simulink library "HEMERO"  (Simulink 3.00)
values from neighbouring files (symbols this model uses):
  K1 = 0.5    [ejh64.m]    (also in ejh65.m)
  K2 = 0.8    [ejh64.m]    (also in ejh65.m)
  x_camino = 0:0.01:10    [ejh64.m]    (also in ejh65.m)
  y_camino = x_camino.^2    [ejh64.m]    (also in ejh65.m)
undefined symbols (not defined in the file or in its folder): magnitude, nonlinear
libraries: simulink_extras x12, HEMERO x9, simulink3 x6, dspstat x4
(part 3 of 9)

== system HEMERO/Robots móviles/Control de robots móviles/Métodos basados en Teoría de Control/Seguimiento de trayectorias ==
  Ejemplos : Subsystem
  Seguimiento de trayectorias (Control lineal con escalado de velocidad) : Subsystem  mask(Seguimiento de trayectorias (control lineal y escalado en velocidad)){b=, d=, x_inicial=, y_inicial=, phi_inicial=, x_r_inicial=, y_r_inicial=, phi_r_inicial=}
      mask prompts: b "Parámetro beta:"; d "Parámetro delta:"; x_inicial "Coordenada x inicial del robot:"; y_inicial "Coordenada y inicial del robot:"; phi_inicial "Valor inicial de la orientación del robot (rad):"; x_r_inicial "Coordenada x inicial de la referencia:"; y_r_inicial "Coordenada y inicial de la referencia:"; phi_r_inicial "Orientación inicial de la referencia (rad):"
      mask help:
      | Este bloque permite simular una estrategia de control lineal con "escalado en velocidad" para el seguimiento de trayectorias. A la entrada se dispone de las velocidades lineal y angular de referencia. Se supone un cierto modelo para el vehículo.
      | El usuario puede modificar este bloque para introducir como referencia las coordenadas (x,y) y la orientación deseadas.
  Seguimiento de trayectorias (Control lineal) : Subsystem  mask(Seguimiento de trayectorias empleando una ley de control lineal){K1=, K2=, K3=, x_inicial=, y_inicial=, phi_inicial=, x_r_inicial=, y_r_inicial=, phi_r_inicial=}
      mask prompts: K1 "Parámetro K1:"; K2 "Parámetro K2:"; K3 "Parámetro K3:"; x_inicial "Coordenada x inicial del robot:"; y_inicial "Coordenada y inicial del robot:"; phi_inicial "Valor inicial de la orientación del robot (rad):"; x_r_inicial "Coordenada x inicial de la referencia:"; y_r_inicial "Coordenada y inicial de la referencia:"; phi_r_inicial "Orientación inicial de la referencia (rad):"
      mask help:
      | Este bloque permite simular una estrategia de control lineal para el seguimiento de trayectorias. A la entrada se dispone de las velocidades lineal y angular de referencia. Se supone un cierto modelo para el vehículo.
      | El usuario puede modificar este bloque para introducir como referencia las coordenadas (x,y) y la orientación deseadas.
  Seguimiento de trayectorias (Control no lineal) : Subsystem  mask(Seguimiento de trayectorias empleando una ley de control no lineal){b=, d=, K2=, x_inicial=, y_inicial=, phi_inicial=, x_r_inicial=, y_r_inicial=, phi_r_inicial=}
      mask prompts: b "Parámetro beta:"; d "Parámetro delta:"; K2 "Parámetro K2:"; x_inicial "Coordenada x inicial del robot:"; y_inicial "Coordenada y inicial del robot:"; phi_inicial "Valor inicial de la orientación del robot (rad):"; x_r_inicial "Coordenada x inicial de la referencia:"; y_r_inicial "Coordenada y inicial de la referencia:"; phi_r_inicial "Orientación inicial de la referencia (rad):"
      mask help:
      | Este bloque permite simular una estrategia de control no lineal para el seguimiento de trayectorias. A la entrada se dispone de las velocidades lineal y angular de referencia. Se supone un cierto modelo para el vehículo.
      | El usuario puede modificar este bloque para introducir como referencia las coordenadas (x,y) y la orientación deseadas.

== system HEMERO/Robots móviles/Modelos cinemáticos inversos/Modelo inverso Bicicleta/Cálculo de phi ==
  x ' : Inport  Port=1  PortWidth=-1  SampleTime=-1  DataType=auto
      settings: SignalType=auto
  y ' : Inport  Port=2  PortWidth=-1  SampleTime=-1  DataType=auto
      settings: SignalType=auto
  MATLAB Fcn : MATLABFcn  MATLABFcn=auxinv  OutputWidth=1  OutputSignalType=auto
  Mux : Mux  Inputs=2
      settings: DisplayOption=none
  phi : Outport  Port=1
  wires:
  Mux/1 -> MATLAB Fcn/1
  y '/1 -> Mux/2
  x '/1 -> Mux/1
  MATLAB Fcn/1 -> phi/1

== system HEMERO/Robots móviles/Modelos cinemáticos inversos/Modelo inverso Config. Síncrona/Cálculo de phi ==
  x ' : Inport  Port=1  PortWidth=-1  SampleTime=-1  DataType=auto
      settings: SignalType=auto
  y ' : Inport  Port=2  PortWidth=-1  SampleTime=-1  DataType=auto
      settings: SignalType=auto
  MATLAB Fcn : MATLABFcn  MATLABFcn=auxinv  OutputWidth=1  OutputSignalType=auto
  Mux : Mux  Inputs=2
      settings: DisplayOption=none
  phi : Outport  Port=1
  wires:
  Mux/1 -> MATLAB Fcn/1
  y '/1 -> Mux/2
  x '/1 -> Mux/1
  MATLAB Fcn/1 -> phi/1

== system HEMERO/Robots móviles/Modelos cinemáticos inversos/Modelo inverso Guiado Diferencial/Cálculo de phi ==
  x ' : Inport  Port=1  PortWidth=-1  SampleTime=-1  DataType=auto
      settings: SignalType=auto
  y ' : Inport  Port=2  PortWidth=-1  SampleTime=-1  DataType=auto
      settings: SignalType=auto
  MATLAB Fcn : MATLABFcn  MATLABFcn=auxinv  OutputWidth=1  OutputSignalType=auto
  Mux : Mux  Inputs=2
      settings: DisplayOption=none
  phi : Outport  Port=1
  wires:
  Mux/1 -> MATLAB Fcn/1
  y '/1 -> Mux/2
  x '/1 -> Mux/1
  MATLAB Fcn/1 -> phi/1

== system HEMERO/Robots móviles/Modelos cinemáticos inversos/Modelo inverso Triciclo Clasico/Cálculo de phi ==
  x ' : Inport  Port=1  PortWidth=-1  SampleTime=-1  DataType=auto
      settings: SignalType=auto
  y ' : Inport  Port=2  PortWidth=-1  SampleTime=-1  DataType=auto
      settings: SignalType=auto
  MATLAB Fcn : MATLABFcn  MATLABFcn=auxinv  OutputWidth=1  OutputSignalType=auto
  Mux : Mux  Inputs=2
      settings: DisplayOption=none
  phi : Outport  Port=1
  wires:
  MATLAB Fcn/1 -> phi/1
  x '/1 -> Mux/1
  y '/1 -> Mux/2
  Mux/1 -> MATLAB Fcn/1

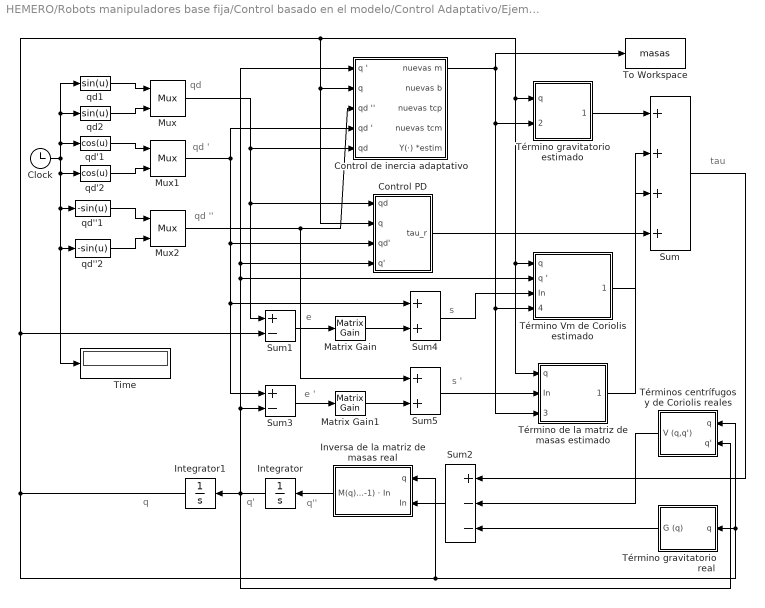
== system HEMERO/Robots manipuladores base fija/Control basado en el modelo/Control Adaptativo/Ejemplos/Ejemplo H.5.5 ==
  note: q''
  note: q'
  note: q
  note: tau
  note: e
  note: e '
  note: s
  note: s '
  note: qd
  note: qd '
  note: qd ''
  Clock : Clock
      settings: DisplayTime=off  Decimation=10
  Control PD : Subsystem  mask(Controlador PD){A=[2.5 0;0 2.5], Kv=[10 0;0 10]}
      mask prompts: A "Introduzca la matriz A:"; Kv "Introduzca la matriz Kv:"
      mask help: Calcula el par tau_r correspondiente a la técnica del par computado usando un controlador PD.
  Control de inercia adaptativo : Subsystem  mask(Técnica del par computado con control adaptativo){dyn=[0 0 0 0 0 30 1 0 0 0 0 0 0 0 0 0 1 0 0 0;0 1 0 0 0 100 1 0 0 0 0 0 0 0 0 0 1 0 0 0], gamma=[20 0 zeros(1,6); 0 20 zeros(1,6); zeros(6,8)], a=[2.5 0;0 2.5], grav=[0 -9.81 0], m_inicial=[30 100], b_inicial=[0 0], tcp_inicial=[0 0], tcm_inicial=[0 0]}
      mask prompts: dyn "Matriz de parámetros cinemáticos y dinámicos:"; gamma "Matriz gamma:"; a "Matriz A:"; grav "Vector aceleración de la gravedad:"; m_inicial "Estimaciones de las masas:"; b_inicial "Estimaciones de las fricciones viscosas:"; tcp_inicial "Estimaciones de las fricciones de Coulomb (rotación +):"; tcm_inicial "Estimaciones de las fricciones de Coulomb (rotación -):"
  Integrator : Integrator  Orientation=left  ExternalReset=none  InitialConditionSource=internal  InitialCondition=[0;0]  LimitOutput=off  UpperSaturationLimit=inf  LowerSaturationLimit=-inf  ShowSaturationPort=off  ShowStatePort=off  AbsoluteTolerance=auto
  Integrator1 : Integrator  Orientation=left  ExternalReset=none  InitialConditionSource=internal  InitialCondition=[0; 0]  LimitOutput=off  UpperSaturationLimit=inf  LowerSaturationLimit=-inf  ShowSaturationPort=off  ShowStatePort=off  AbsoluteTolerance=auto
  Inversa de la matriz de masas real : Subsystem  Orientation=left  mask(Inversa de la matriz de masas){dyn=[0 0 0 0 0 0.8 1 0 0 0 0 0 0 0 0 0 1 0 0 0;0 1 0 0 0 2.3 1 0 0 0 0 0 0 0 0 0 1 0 0 0]}
      mask prompts: dyn "Matriz de parámetros cinemáticos y dinámicos:"
      mask help: Este bloque calcula el producto de la inversa de la matriz de masas por el vector columna In que se le pasa como entrada.
  Matrix Gain : simulink3/Math/Matrix Gain  K=[2.5 0;0 2.5]
  Matrix Gain1 : simulink3/Math/Matrix Gain  K=[2.5 0;0 2.5]
  Mux : Mux  Inputs=2
      settings: DisplayOption=none
  Mux1 : Mux  Inputs=2
      settings: DisplayOption=none
  Mux2 : Mux  Inputs=2
      settings: DisplayOption=none
  Sum : Sum  Inputs=++++  SaturateOnIntegerOverflow=on
  Sum1 : Sum  Inputs=+-  SaturateOnIntegerOverflow=on
  Sum2 : Sum  Orientation=left  Inputs=+--  SaturateOnIntegerOverflow=on
  Sum3 : Sum  Inputs=+-  SaturateOnIntegerOverflow=on
  Sum4 : Sum  Inputs=++  SaturateOnIntegerOverflow=on
  Sum5 : Sum  Inputs=++  SaturateOnIntegerOverflow=on
  Time : Display
      settings: Format=short
  To Workspace : ToWorkspace  VariableName=masas  SampleTime=-1  SaveFormat=Matrix
  Término gravitatorio estimado : Subsystem  mask(Término gravitatorio estimado){dyn=[0 0 0 0 0 30 1 0 0 0 0 0 0 0 0 0 1 0 0 0;0 1 0 0 0 100 1 0 0 0 0 0 0 0 0 0 1 0 0 0], grav=[0 -9.81 0]}
      mask prompts: dyn "Matriz inicial de parámetros cinemáticos y dinámicos:"; grav "Vector aceleración de la gravedad:"
      mask help: Este bloque calcula el par correspondiente al término gravitatorio. Dispone de una entrada para proporcionarle las estimaciones de las masas en cada instante.
      mask Display:
      | plot([0.05 0.95],[0.05 0.95])
      | plot([0.8 0.95],[0.7 0.95])
      | plot([0.7 0.95],[0.8 0.95])
  Término gravitatorio real : Subsystem  Orientation=left  mask(Término gravitatorio){dyn=[0 0 0 0 0 0.8 1 0 0 0 0 0 0 0 0 0 1 0 0 0;0 1 0 0 0 2.3 1 0 0 0 0 0 0 0 0 0 1 0 0 0], grav=[0 -9.81 0]}
      mask prompts: dyn "Matriz de parámetros cinemáticos y dinámicos:"; grav "Vector aceleración de la gravedad:"
      mask help: Este bloque calcula el par correspondiente al término gravitatorio.
  Término Vm de Coriolis estimado : Subsystem  mask(Término estimado asociado a la matriz de masas){dyn=[0 0 0 0 0 30 1 0 0 0 0 0 0 0 0 0 1 0 0 0;0 1 0 0 0 100 1 0 0 0 0 0 0 0 0 0 1 0 0 0]}
      mask prompts: dyn "Matriz inicial de parámetros cinemáticos y dinámicos:"
      mask help: Este bloque calcula el par correspondiente al término en el que aparece la matriz de masas. Dispone de una entrada para proporcionarle las estimaciones de las masas en cada instante.
      mask Display:
      | plot([0.05 0.95],[0.05 0.95])
      | plot([0.8 0.95],[0.7 0.95])
      | plot([0.7 0.95],[0.8 0.95])
  Término de la matriz de masas estimado : Subsystem  mask(Término estimado asociado a la matriz de masas){dyn=[0 0 0 0 0 30 1 0 0 0 0 0 0 0 0 0 1 0 0 0;0 1 0 0 0 100 1 0 0 0 0 0 0 0 0 0 1 0 0 0]}
      mask prompts: dyn "Matriz inicial de parámetros cinemáticos y dinámicos:"
      mask help: Este bloque calcula el par correspondiente al término en el que aparece la matriz de masas. Dispone de una entrada para proporcionarle las estimaciones de las masas en cada instante.
      mask Display:
      | plot([0.05 0.95],[0.05 0.95])
      | plot([0.8 0.95],[0.7 0.95])
      | plot([0.7 0.95],[0.8 0.95])
  Términos centrífugos y de Coriolis reales : Subsystem  Orientation=left  mask(Términos centrífugos y de Coriolis){dyn=[0 0 0 0 0 0.8 1 0 0 0 0 0 0 0 0 0 1 0 0 0;0 1 0 0 0 2.3 1 0 0 0 0 0 0 0 0 0 1 0 0 0]}
      mask prompts: dyn "Matriz de parámetros cinemáticos y dinámicos:"
      mask help: Este bloque calcula el par correspondiente a los términos centrífugos y de Coriolis.
  qd''1 : Fcn  Expr=-sin(u)
  qd''2 : Fcn  Expr=-sin(u)
  qd'1 : Fcn  Expr=cos(u)
  qd'2 : Fcn  Expr=cos(u)
  qd1 : Fcn  Expr=sin(u)
  qd2 : Fcn  Expr=sin(u)
  wires:
  qd''2/1 -> Mux2/2
  qd''1/1 -> Mux2/1
  qd'2/1 -> Mux1/2
  qd'1/1 -> Mux1/1
  qd2/1 -> Mux/2
  qd1/1 -> Mux/1
  Control PD/1(tau_r) -> Sum/4
  Término Vm de Coriolis estimado/1(Vm (q,q')·In) -> Sum/2
  Término de la matriz de masas estimado/1(M (q)·In) -> Sum/3
  Clock/1 -> qd''1/1, qd''2/1, Time/1, qd'2/1, qd'1/1, qd1/1, qd2/1
  Mux1/1 -> Control PD/3(qd'), Sum3/1, Sum4/1, Control de inercia adaptativo/4(qd ')
  Sum1/1 -> Matrix Gain/1
  Sum3/1 -> Matrix Gain1/1
  Matrix Gain1/1 -> Sum5/2
  Matrix Gain/1 -> Sum4/2
  Sum5/1 -> Término de la matriz de masas estimado/2(In)
  Sum4/1 -> Término Vm de Coriolis estimado/3(In)
  Término gravitatorio estimado/1(G (q)) -> Sum/1
  Integrator/1 -> Integrator1/1, Términos centrífugos y de Coriolis reales/2(q'), Control de inercia adaptativo/1(q '), Control PD/4(q'), Término Vm de Coriolis estimado/2(q '), Sum3/2
  Sum2/1 -> Inversa de la matriz de masas real/2(In)
  Integrator1/1 -> Inversa de la matriz de masas real/1(q), Términos centrífugos y de Coriolis reales/1(q), Término gravitatorio real/1(q), Sum1/2, Control PD/2(q), Control de inercia adaptativo/2(q), Término gravitatorio estimado/1(q), Término Vm de Coriolis estimado/1(q), Término de la matriz de masas estimado/1(q)
  Inversa de la matriz de masas real/1(M(q)^(-1) · In) -> Integrator/1
  Sum/1 -> Sum2/1
  Mux/1 -> Control de inercia adaptativo/5(qd), Sum1/1, Control PD/1(qd)
  Mux2/1 -> Control de inercia adaptativo/3(qd ''), Sum5/1
  Términos centrífugos y de Coriolis reales/1(V (q,q')) -> Sum2/2
  Término gravitatorio real/1(G (q)) -> Sum2/3
  Control de inercia adaptativo/1(nuevas m) -> Término gravitatorio estimado/2(nuevas m), Término de la matriz de masas estimado/3(nuevas m), Término Vm de Coriolis estimado/4(nuevas m), To Workspace/1

== system HEMERO/Robots manipuladores base fija/Control basado en el modelo/Control con aprendizaje/Ejemplos/Ejemplo H.5.1 ==
  note: tau
  note: qd '
  Clock : Clock
      settings: DisplayTime=off  Decimation=10
  Control PD : Subsystem  mask(Controlador PD){Kp=[625 0;0 625], Kv=[50 0;0 50]}
      mask prompts: Kp "Introduzca la matriz Kp:"; Kv "Introduzca la matriz Kv:"
      mask help: Calcula el par tau_r correspondiente a la técnica del par computado usando un controlador PD.
  Modelo del robot : Subsystem  Orientation=left  mask(Trayectorias articulares){dyn=[0 0 0 0 0 0.8 1 0 0 0 0 0 0 0 0 0 1 10 0 0;0 1 0 0 0 2.3 1 0 0 0 0 0 0 0 0 0 1 5 0 0], grav=[0 -9.81 0], inivel=[0 0], inipos=[0 0]}
      mask prompts: dyn "Matriz de parámetros cinemáticos y dinámicos:"; grav "Vector aceleración de la gravedad:"; inivel "Velocidades articulares iniciales:"; inipos "Posiciones articulares iniciales:"
      mask help: Se calculan las trayectorias articulares (posiciones, velocidades y aceleraciones articulares) a partir de los pares aplicados al manipulador.
  Mux : Mux  Inputs=2
      settings: DisplayOption=none
  Mux1 : Mux  Inputs=2
      settings: DisplayOption=none
  Mux2 : Mux  Inputs=2
      settings: DisplayOption=none
  Par realimentado aprendido : Subsystem  mask{dyn=[0 0 0 0 0 0.8 1 0 0 0 0 0 0 0 0 0 1 0 0 0;0 1 0 0 0 2.3 1 0 0 0 0 0 0 0 0 0 1 0 0 0], Kp=625*eye(2), Kv=50*eye(2), mu=[3 0; 0 3], tfinal=2.5}
      mask prompts: dyn "Matriz de parámetros cinemáticos y dinámicos:"; Kp "Matriz Kp:"; Kv "Matriz Kv:"; mu "Constante mu:"; tfinal "Tiempo final de la simulación:"
  Sum : Sum  Inputs=++++  SaturateOnIntegerOverflow=on
  To Workspace : ToWorkspace  VariableName=q  SampleTime=-1  SaveFormat=Matrix
  Término de la matriz de masas : Subsystem  mask(Término asociado a la matriz de masas){dyn=[0 0 0 0 0 0.8 1 0 0 0 0 0 0 0 0 0 1 0 0 0;0 1 0 0 0 2.3 1 0 0 0 0 0 0 0 0 0 1 0 0 0]}
      mask prompts: dyn "Matriz de parámetros cinemáticos y dinámicos:"
      mask help: Este bloque calcula el par correspondiente al término en el que aparece la matriz de masas.
  Términos gravitatorios : Subsystem  mask(Término gravitatorio){dyn=[0 0 0 0 0 0.8 1 0 0 0 0 0 0 0 0 0 1 0 0 0;0 1 0 0 0 2.3 1 0 0 0 0 0 0 0 0 0 1 0 0 0], grav=[0 -9.81 0]}
      mask prompts: dyn "Matriz de parámetros cinemáticos y dinámicos:"; grav "Vector aceleración de la gravedad:"
      mask help: Este bloque calcula el par correspondiente al término gravitatorio.
  Términos centrífugos y de Coriolis : Subsystem  mask(Términos centrífugos y de Coriolis){dyn=[0 0 0 0 0 0.8 1 0 0 0 0 0 0 0 0 0 1 0 0 0;0 1 0 0 0 2.3 1 0 0 0 0 0 0 0 0 0 1 0 0 0]}
      mask prompts: dyn "Matriz de parámetros cinemáticos y dinámicos:"
      mask help: Este bloque calcula el par correspondiente a los términos centrífugos y de Coriolis.
  qd : Fcn  Expr=u
  qd '' : Fcn  Expr=0
  qd'1 : Fcn  Expr=1
  wires:
  Mux/1 -> Control PD/1(qd), Par realimentado aprendido/5(qd)
  Clock/1 -> qd/1, qd'1/1, qd ''/1
  Mux2/1 -> Control PD/5(qd''), Par realimentado aprendido/1(qd '')
  Mux1/1 -> Control PD/3(qd'), Par realimentado aprendido/3(qd ')
  qd/1 -> Mux/1, Mux/2
  qd'1/1 -> Mux1/1, Mux1/2
  qd ''/1 -> Mux2/1, Mux2/2
  Término de la matriz de masas/1(M (q)·In) -> Sum/2
  Términos centrífugos y de Coriolis/1(V (q,q')) -> Sum/3
  Términos gravitatorios/1(G (q)) -> Sum/1
  Control PD/1(tau_r) -> Término de la matriz de masas/2(In)
  Modelo del robot/2(q') -> Términos centrífugos y de Coriolis/2(q'), Control PD/4(q'), Par realimentado aprendido/4(q ')
  Modelo del robot/1(q) -> To Workspace/1, Control PD/2(q), Par realimentado aprendido/6(q), Términos centrífugos y de Coriolis/1(q), Término de la matriz de masas/1(q), Términos gravitatorios/1(q)
  Modelo del robot/3(q'') -> Par realimentado aprendido/2(q '')
  Sum/1 -> Modelo del robot/1(tau)
  Par realimentado aprendido/1(gamma (k)) -> Sum/4

== system HEMERO/Robots manipuladores base fija/Control basado en el modelo/Control con aprendizaje/Par realimentado aprendido/Término de la matriz de masas estimado ==
  q : Inport  Port=1  PortWidth=-1  SampleTime=-1  DataType=auto
      settings: SignalType=auto
  In : Inport  Port=2  PortWidth=-1  SampleTime=-1  DataType=auto
      settings: SignalType=auto
  Masas : S-Function  FunctionName=sinertia  Parameters=dyn  PortCounts=[]  SFunctionModules=''
  Mux : Mux  Inputs=2
      settings: DisplayOption=none
  M (q)·In : Outport  Port=1  InitialOutput=0
  wires:
  Mux/1 -> Masas/1
  q/1 -> Mux/1
  In/1 -> Mux/2
  Masas/1 -> M (q)·In/1

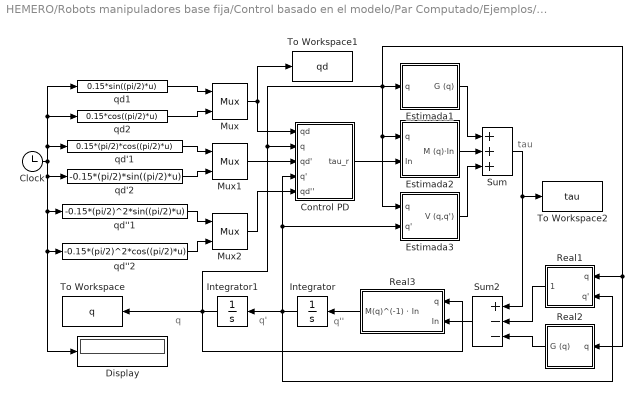
== system HEMERO/Robots manipuladores base fija/Control basado en el modelo/Par Computado/Ejemplos/Ejemplo H.5.2 ==
  note: tau
  note: q
  note: q'
  note: q''
  Clock : Clock
      settings: DisplayTime=off  Decimation=10
  Control PD : Subsystem  mask(Controlador PD){Kp=[25 0;0 25], Kv=[10 0;0 10]}
      mask prompts: Kp "Introduzca la matriz Kp:"; Kv "Introduzca la matriz Kv:"
      mask help: Calcula el par tau_r correspondiente a la técnica del par computado usando un controlador PD.
  Display : Display
      settings: Format=short
  Estimada1 : Subsystem  mask(Término gravitatorio){dyn=[0 0 0 0 0 2 3 0 0 0 0 0 0 0 0 0 1 0 0 0;0 3 0 0 0 1 1 0 0 0 0 0 0 0 0 0 1 0 0 0], grav=[0 -9.81 0]}
      mask prompts: dyn "Matriz de parámetros cinemáticos y dinámicos:"; grav "Vector aceleración de la gravedad:"
      mask help: Este bloque calcula el par correspondiente al término gravitatorio.
  Estimada2 : Subsystem  mask(Término asociado a la matriz de masas){dyn=[0 0 0 0 0 2 3 0 0 0 0 0 0 0 0 0 1 0 0 0;0 3 0 0 0 1 1 0 0 0 0 0 0 0 0 0 1 0 0 0]}
      mask prompts: dyn "Matriz de parámetros cinemáticos y dinámicos:"
      mask help: Este bloque calcula el par correspondiente al término en el que aparece la matriz de masas.
  Estimada3 : Subsystem  mask(Términos centrífugos y de Coriolis){dyn=[0 0 0 0 0 2 3 0 0 0 0 0 0 0 0 0 1 0 0 0;0 3 0 0 0 1 1 0 0 0 0 0 0 0 0 0 1 0 0 0]}
      mask prompts: dyn "Matriz de parámetros cinemáticos y dinámicos:"
      mask help: Este bloque calcula el par correspondiente a los términos centrífugos y de Coriolis.
  Integrator : Integrator  Orientation=left  ExternalReset=none  InitialConditionSource=internal  InitialCondition=[0;0]  LimitOutput=off  UpperSaturationLimit=inf  LowerSaturationLimit=-inf  ShowSaturationPort=off  ShowStatePort=off  AbsoluteTolerance=auto
  Integrator1 : Integrator  Orientation=left  ExternalReset=none  InitialConditionSource=internal  InitialCondition=[0; 0]  LimitOutput=off  UpperSaturationLimit=inf  LowerSaturationLimit=-inf  ShowSaturationPort=off  ShowStatePort=off  AbsoluteTolerance=auto
  Mux : Mux  Inputs=2
      settings: DisplayOption=none
  Mux1 : Mux  Inputs=2
      settings: DisplayOption=none
  Mux2 : Mux  Inputs=2
      settings: DisplayOption=none
  Real1 : Subsystem  Orientation=left  mask(Términos centrífugos y de Coriolis){dyn=[0 0 0 0 0 2 3 0 0 0 0 0 0 0 0 0 1 0 0 0;0 3 0 0 0 1 1 0 0 0 0 0 0 0 0 0 1 0 0 0]}
      mask prompts: dyn "Matriz de parámetros cinemáticos y dinámicos:"
      mask help: Este bloque calcula el par correspondiente a los términos centrífugos y de Coriolis.
  Real2 : Subsystem  Orientation=left  mask(Término gravitatorio){dyn=[0 0 0 0 0 2 3 0 0 0 0 0 0 0 0 0 1 0 0 0;0 3 0 0 0 1 1 0 0 0 0 0 0 0 0 0 1 0 0 0], grav=[0 -9.81 0]}
      mask prompts: dyn "Matriz de parámetros cinemáticos y dinámicos:"; grav "Vector aceleración de la gravedad:"
      mask help: Este bloque calcula el par correspondiente al término gravitatorio.
  Real3 : Subsystem  Orientation=left  mask(Inversa de la matriz de masas){dyn=[0 0 0 0 0 2 3 0 0 0 0 0 0 0 0 0 1 0 0 0;0 3 0 0 0 1 1 0 0 0 0 0 0 0 0 0 1 0 0 0]}
      mask prompts: dyn "Matriz de parámetros cinemáticos y dinámicos:"
      mask help: Este bloque calcula el producto de la inversa de la matriz de masas por el vector columna In que se le pasa como entrada.
  Sum : Sum  Inputs=+++  SaturateOnIntegerOverflow=on
  Sum2 : Sum  Orientation=left  Inputs=+--  SaturateOnIntegerOverflow=on
  To Workspace : ToWorkspace  VariableName=q  SampleTime=-1  SaveFormat=Matrix
  To Workspace1 : ToWorkspace  VariableName=qd  SampleTime=-1  SaveFormat=Matrix
  To Workspace2 : ToWorkspace  VariableName=tau  SampleTime=-1  SaveFormat=Matrix
  qd''1 : Fcn  Expr=-0.15*(pi/2)^2*sin((pi/2)*u)
  qd''2 : Fcn  Expr=-0.15*(pi/2)^2*cos((pi/2)*u)
  qd'1 : Fcn  Expr=0.15*(pi/2)*cos((pi/2)*u)
  qd'2 : Fcn  Expr=-0.15*(pi/2)*sin((pi/2)*u)
  qd1 : Fcn  Expr=0.15*sin((pi/2)*u)
  qd2 : Fcn  Expr=0.15*cos((pi/2)*u)
  wires:
  Sum/1 -> To Workspace2/1, Sum2/1
  Mux/1 -> To Workspace1/1, Control PD/1(qd)
  Control PD/1(tau_r) -> Estimada2/2(In)
  Clock/1 -> qd'1/1, qd2/1, qd1/1, qd'2/1, qd''1/1, qd''2/1, Display/1
  qd1/1 -> Mux/1
  qd2/1 -> Mux/2
  qd'1/1 -> Mux1/1
  qd'2/1 -> Mux1/2
  qd''1/1 -> Mux2/1
  qd''2/1 -> Mux2/2
  Mux1/1 -> Control PD/3(qd')
  Mux2/1 -> Control PD/5(qd'')
  Estimada2/1(M (q)·In) -> Sum/2
  Estimada1/1(G (q)) -> Sum/1
  Estimada3/1(V (q,q')) -> Sum/3
  Real2/1(G (q)) -> Sum2/3
  Real1/1(V (q,q')) -> Sum2/2
  Sum2/1 -> Real3/2(In)
  Integrator/1 -> Integrator1/1, Control PD/4(q'), Estimada3/2(q'), Real1/2(q')
  Integrator1/1 -> Control PD/2(q), Estimada1/1(q), Estimada2/1(q), Estimada3/1(q), Real1/1(q), Real2/1(q), To Workspace/1, Real3/1(q)
  Real3/1(M(q)^(-1) · In) -> Integrator/1

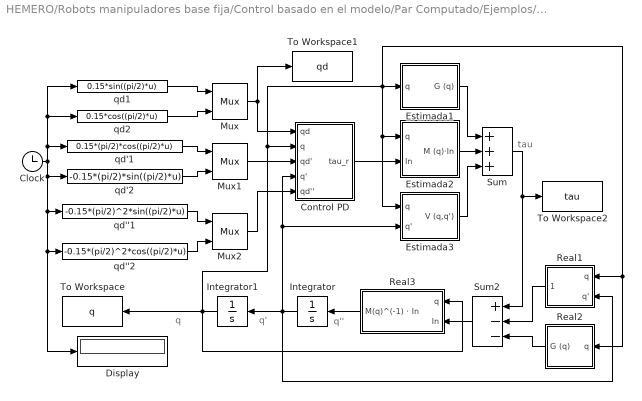
== system HEMERO/Robots manipuladores base fija/Control basado en el modelo/Par Computado/Ejemplos/Ejemplo H.5.3 ==
  note: tau
  note: q
  note: q'
  note: q''
  Clock : Clock
      settings: DisplayTime=off  Decimation=10
  Control PD : Subsystem  mask(Controlador PD){Kp=[25 0;0 25], Kv=[10 0;0 10]}
      mask prompts: Kp "Introduzca la matriz Kp:"; Kv "Introduzca la matriz Kv:"
      mask help: Calcula el par tau_r correspondiente a la técnica del par computado usando un controlador PD.
  Display : Display
      settings: Format=short
  Estimada1 : Subsystem  mask(Término gravitatorio){dyn=[0 0 0 0 0 2.1 3 0 0 0 0 0 0 0 0 0 1 0 0 0;0 3 0 0 0 0.9 1 0 0 0 0 0 0 0 0 0 1 0 0 0], grav=[0 -9.81 0]}
      mask prompts: dyn "Matriz de parámetros cinemáticos y dinámicos:"; grav "Vector aceleración de la gravedad:"
      mask help: Este bloque calcula el par correspondiente al término gravitatorio.
  Estimada2 : Subsystem  mask(Término asociado a la matriz de masas){dyn=[0 0 0 0 0 2.1 3 0 0 0 0 0 0 0 0 0 1 0 0 0;0 3 0 0 0 0.9 1 0 0 0 0 0 0 0 0 0 1 0 0 0]}
      mask prompts: dyn "Matriz de parámetros cinemáticos y dinámicos:"
      mask help: Este bloque calcula el par correspondiente al término en el que aparece la matriz de masas.
  Estimada3 : Subsystem  mask(Términos centrífugos y de Coriolis){dyn=[0 0 0 0 0 2.1 3 0 0 0 0 0 0 0 0 0 1 0 0 0;0 3 0 0 0 0.9 1 0 0 0 0 0 0 0 0 0 1 0 0 0]}
      mask prompts: dyn "Matriz de parámetros cinemáticos y dinámicos:"
      mask help: Este bloque calcula el par correspondiente a los términos centrífugos y de Coriolis.
  Integrator : Integrator  Orientation=left  ExternalReset=none  InitialConditionSource=internal  InitialCondition=[0;0]  LimitOutput=off  UpperSaturationLimit=inf  LowerSaturationLimit=-inf  ShowSaturationPort=off  ShowStatePort=off  AbsoluteTolerance=auto
  Integrator1 : Integrator  Orientation=left  ExternalReset=none  InitialConditionSource=internal  InitialCondition=[0; 0]  LimitOutput=off  UpperSaturationLimit=inf  LowerSaturationLimit=-inf  ShowSaturationPort=off  ShowStatePort=off  AbsoluteTolerance=auto
  Mux : Mux  Inputs=2
      settings: DisplayOption=none
  Mux1 : Mux  Inputs=2
      settings: DisplayOption=none
  Mux2 : Mux  Inputs=2
      settings: DisplayOption=none
  Real1 : Subsystem  Orientation=left  mask(Términos centrífugos y de Coriolis){dyn=[0 0 0 0 0 2 3 0 0 0 0 0 0 0 0 0 1 0 0 0;0 3 0 0 0 1 1 0 0 0 0 0 0 0 0 0 1 0 0 0]}
      mask prompts: dyn "Matriz de parámetros cinemáticos y dinámicos:"
      mask help: Este bloque calcula el par correspondiente a los términos centrífugos y de Coriolis.
  Real2 : Subsystem  Orientation=left  mask(Término gravitatorio){dyn=[0 0 0 0 0 2 3 0 0 0 0 0 0 0 0 0 1 0 0 0;0 3 0 0 0 1 1 0 0 0 0 0 0 0 0 0 1 0 0 0], grav=[0 -9.81 0]}
      mask prompts: dyn "Matriz de parámetros cinemáticos y dinámicos:"; grav "Vector aceleración de la gravedad:"
      mask help: Este bloque calcula el par correspondiente al término gravitatorio.
  Real3 : Subsystem  Orientation=left  mask(Inversa de la matriz de masas){dyn=[0 0 0 0 0 2 3 0 0 0 0 0 0 0 0 0 1 0 0 0;0 3 0 0 0 1 1 0 0 0 0 0 0 0 0 0 1 0 0 0]}
      mask prompts: dyn "Matriz de parámetros cinemáticos y dinámicos:"
      mask help: Este bloque calcula el producto de la inversa de la matriz de masas por el vector columna In que se le pasa como entrada.
  Sum : Sum  Inputs=+++  SaturateOnIntegerOverflow=on
  Sum2 : Sum  Orientation=left  Inputs=+--  SaturateOnIntegerOverflow=on
  To Workspace : ToWorkspace  VariableName=q  SampleTime=-1  SaveFormat=Matrix
  To Workspace1 : ToWorkspace  VariableName=qd  SampleTime=-1  SaveFormat=Matrix
  To Workspace2 : ToWorkspace  VariableName=tau  SampleTime=-1  SaveFormat=Matrix
  qd''1 : Fcn  Expr=-0.15*(pi/2)^2*sin((pi/2)*u)
  qd''2 : Fcn  Expr=-0.15*(pi/2)^2*cos((pi/2)*u)
  qd'1 : Fcn  Expr=0.15*(pi/2)*cos((pi/2)*u)
  qd'2 : Fcn  Expr=-0.15*(pi/2)*sin((pi/2)*u)
  qd1 : Fcn  Expr=0.15*sin((pi/2)*u)
  qd2 : Fcn  Expr=0.15*cos((pi/2)*u)
  wires:
  Sum/1 -> To Workspace2/1, Sum2/1
  Mux/1 -> To Workspace1/1, Control PD/1(qd)
  Control PD/1(tau_r) -> Estimada2/2(In)
  Clock/1 -> qd'1/1, qd2/1, qd1/1, qd'2/1, qd''1/1, qd''2/1, Display/1
  qd1/1 -> Mux/1
  qd2/1 -> Mux/2
  qd'1/1 -> Mux1/1
  qd'2/1 -> Mux1/2
  qd''1/1 -> Mux2/1
  qd''2/1 -> Mux2/2
  Mux1/1 -> Control PD/3(qd')
  Mux2/1 -> Control PD/5(qd'')
  Estimada2/1(M (q)·In) -> Sum/2
  Estimada1/1(G (q)) -> Sum/1
  Estimada3/1(V (q,q')) -> Sum/3
  Real2/1(G (q)) -> Sum2/3
  Real1/1(V (q,q')) -> Sum2/2
  Sum2/1 -> Real3/2(In)
  Integrator/1 -> Integrator1/1, Control PD/4(q'), Estimada3/2(q'), Real1/2(q')
  Integrator1/1 -> Control PD/2(q), Estimada1/1(q), Estimada2/1(q), Estimada3/1(q), Real1/1(q), Real2/1(q), To Workspace/1, Real3/1(q)
  Real3/1(M(q)^(-1) · In) -> Integrator/1

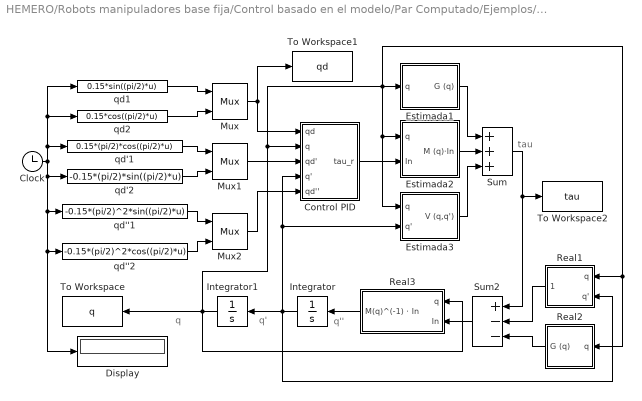
== system HEMERO/Robots manipuladores base fija/Control basado en el modelo/Par Computado/Ejemplos/Ejemplo H.5.4 ==
  note: tau
  note: q
  note: q'
  note: q''
  Clock : Clock
      settings: DisplayTime=off  Decimation=10
  Control PID : Subsystem  mask(Controlador PID){Kp=[25 0;0 25], Kv=[10 0;0 10], Ki=[100 0;0 100]}
      mask prompts: Kp "Introduzca la matriz Kp:"; Kv "Introduzca la matriz Kv:"; Ki "Introduzca la matriz Ki:"
      mask help: Calcula el par tau_r correspondiente a la técnica del par computado usando un controlador PID.
  Display : Display
      settings: Format=short
  Estimada1 : Subsystem  mask(Término gravitatorio){dyn=[0 0 0 0 0 2.1 3 0 0 0 0 0 0 0 0 0 1 0 0 0;0 3 0 0 0 0.9 1 0 0 0 0 0 0 0 0 0 1 0 0 0], grav=[0 -9.81 0]}
      mask prompts: dyn "Matriz de parámetros cinemáticos y dinámicos:"; grav "Vector aceleración de la gravedad:"
      mask help: Este bloque calcula el par correspondiente al término gravitatorio.
  Estimada2 : Subsystem  mask(Término asociado a la matriz de masas){dyn=[0 0 0 0 0 2.1 3 0 0 0 0 0 0 0 0 0 1 0 0 0;0 3 0 0 0 0.9 1 0 0 0 0 0 0 0 0 0 1 0 0 0]}
      mask prompts: dyn "Matriz de parámetros cinemáticos y dinámicos:"
      mask help: Este bloque calcula el par correspondiente al término en el que aparece la matriz de masas.
  Estimada3 : Subsystem  mask(Términos centrífugos y de Coriolis){dyn=[0 0 0 0 0 2.1 3 0 0 0 0 0 0 0 0 0 1 0 0 0;0 3 0 0 0 0.9 1 0 0 0 0 0 0 0 0 0 1 0 0 0]}
      mask prompts: dyn "Matriz de parámetros cinemáticos y dinámicos:"
      mask help: Este bloque calcula el par correspondiente a los términos centrífugos y de Coriolis.
  Integrator : Integrator  Orientation=left  ExternalReset=none  InitialConditionSource=internal  InitialCondition=[0;0]  LimitOutput=off  UpperSaturationLimit=inf  LowerSaturationLimit=-inf  ShowSaturationPort=off  ShowStatePort=off  AbsoluteTolerance=auto
  Integrator1 : Integrator  Orientation=left  ExternalReset=none  InitialConditionSource=internal  InitialCondition=[0; 0]  LimitOutput=off  UpperSaturationLimit=inf  LowerSaturationLimit=-inf  ShowSaturationPort=off  ShowStatePort=off  AbsoluteTolerance=auto
  Mux : Mux  Inputs=2
      settings: DisplayOption=none
  Mux1 : Mux  Inputs=2
      settings: DisplayOption=none
  Mux2 : Mux  Inputs=2
      settings: DisplayOption=none
  Real1 : Subsystem  Orientation=left  mask(Términos centrífugos y de Coriolis){dyn=[0 0 0 0 0 2 3 0 0 0 0 0 0 0 0 0 1 0 0 0;0 3 0 0 0 1 1 0 0 0 0 0 0 0 0 0 1 0 0 0]}
      mask prompts: dyn "Matriz de parámetros cinemáticos y dinámicos:"
      mask help: Este bloque calcula el par correspondiente a los términos centrífugos y de Coriolis.
  Real2 : Subsystem  Orientation=left  mask(Término gravitatorio){dyn=[0 0 0 0 0 2 3 0 0 0 0 0 0 0 0 0 1 0 0 0;0 3 0 0 0 1 1 0 0 0 0 0 0 0 0 0 1 0 0 0], grav=[0 -9.81 0]}
      mask prompts: dyn "Matriz de parámetros cinemáticos y dinámicos:"; grav "Vector aceleración de la gravedad:"
      mask help: Este bloque calcula el par correspondiente al término gravitatorio.
  Real3 : Subsystem  Orientation=left  mask(Inversa de la matriz de masas){dyn=[0 0 0 0 0 2 3 0 0 0 0 0 0 0 0 0 1 0 0 0;0 3 0 0 0 1 1 0 0 0 0 0 0 0 0 0 1 0 0 0]}
      mask prompts: dyn "Matriz de parámetros cinemáticos y dinámicos:"
      mask help: Este bloque calcula el producto de la inversa de la matriz de masas por el vector columna In que se le pasa como entrada.
  Sum : Sum  Inputs=+++  SaturateOnIntegerOverflow=on
  Sum2 : Sum  Orientation=left  Inputs=+--  SaturateOnIntegerOverflow=on
  To Workspace : ToWorkspace  VariableName=q  SampleTime=-1  SaveFormat=Matrix
  To Workspace1 : ToWorkspace  VariableName=qd  SampleTime=-1  SaveFormat=Matrix
  To Workspace2 : ToWorkspace  VariableName=tau  SampleTime=-1  SaveFormat=Matrix
  qd''1 : Fcn  Expr=-0.15*(pi/2)^2*sin((pi/2)*u)
  qd''2 : Fcn  Expr=-0.15*(pi/2)^2*cos((pi/2)*u)
  qd'1 : Fcn  Expr=0.15*(pi/2)*cos((pi/2)*u)
  qd'2 : Fcn  Expr=-0.15*(pi/2)*sin((pi/2)*u)
  qd1 : Fcn  Expr=0.15*sin((pi/2)*u)
  qd2 : Fcn  Expr=0.15*cos((pi/2)*u)
  wires:
  Sum/1 -> To Workspace2/1, Sum2/1
  Mux/1 -> To Workspace1/1, Control PID/1(qd)
  Control PID/1(tau_r) -> Estimada2/2(In)
  Clock/1 -> qd'1/1, qd2/1, qd1/1, qd'2/1, qd''1/1, qd''2/1, Display/1
  qd1/1 -> Mux/1
  qd2/1 -> Mux/2
  qd'1/1 -> Mux1/1
  qd'2/1 -> Mux1/2
  qd''1/1 -> Mux2/1
  qd''2/1 -> Mux2/2
  Mux1/1 -> Control PID/3(qd')
  Mux2/1 -> Control PID/5(qd'')
  Estimada2/1(M (q)·In) -> Sum/2
  Estimada1/1(G (q)) -> Sum/1
  Estimada3/1(V (q,q')) -> Sum/3
  Real2/1(G (q)) -> Sum2/3
  Real1/1(V (q,q')) -> Sum2/2
  Sum2/1 -> Real3/2(In)
  Integrator/1 -> Integrator1/1, Control PID/4(q'), Estimada3/2(q'), Real1/2(q')
  Integrator1/1 -> Control PID/2(q), Estimada1/1(q), Estimada2/1(q), Estimada3/1(q), Real1/1(q), Real2/1(q), To Workspace/1, Real3/1(q)
  Real3/1(M(q)^(-1) · In) -> Integrator/1

== system HEMERO/Robots manipuladores base fija/Modelo Dinámico/Ejemplos/Ejemplo H.4.2/Trayectorias articulares ==
  note: q'
  note: q''
  note: q
  tau : Inport  Port=1  PortWidth=-1  SampleTime=-1  DataType=auto
      settings: SignalType=auto
  Integrator : Integrator  ExternalReset=none  InitialConditionSource=internal  InitialCondition=inivel(:)  LimitOutput=off  UpperSaturationLimit=inf  LowerSaturationLimit=-inf  ShowSaturationPort=off  ShowStatePort=off  AbsoluteTolerance=auto
  Integrator1 : Integrator  ExternalReset=none  InitialConditionSource=internal  InitialCondition=inipos(:)  LimitOutput=off  UpperSaturationLimit=inf  LowerSaturationLimit=-inf  ShowSaturationPort=off  ShowStatePort=off  AbsoluteTolerance=auto
  Inversa de la matriz de masas : Subsystem  mask(Término de Coriolis){dyn=dyn}
      mask prompts: dyn "Matriz de parámetros dinámicos:"
      mask help: Este bloque devuelve el par correspondiente al término de Coriolis.
      mask Help: A este bloque hay que darle tres parámetros: 1) La matriz de parámetros dinámicos del manipulador de acuerdo con el formato que se explica en la sección "dyn" del Apéndice, 2) Un vector columna correspondiente a la aceleración de la gravedad, y 3) Un vector columna correspondiente a las fuerzas externas.
  Modelo de fricciones : Subsystem  mask(Modelo de fricciones (viscosa y de Coriolis)){G=dyn (:,17), b=dyn (:,18), tcp=dyn (:,19), tcm=dyn (:,20)}
      mask prompts: G "Factores de reducción (G):"; b "Fricciones viscosas, referidas al motor:"; tcp "Fricciones de Coulomb (rotación +), referidas al motor:"; tcm "Fricciones de Coulomb (rotación -), referidas al motor:"
      mask help:
      | Este bloque calcula el par correspondiente a la fricciones viscosa y de Coulomb. Para ello se emplea un determinado modelo para dichas fricciones:
      |            B·q' + Tc + ,  si q'>0
      |            B·q' + Tc - ,  si q'<0
      mask Display:
      | disp('B·q'' + Tc + ,  si q''>0\n')
      | disp('\nB·q'' + Tc - ,  si q''<0')
  Sum : Sum  Inputs=+---  SaturateOnIntegerOverflow=on
  Términos gravitatorios : Subsystem  mask(Término de Coriolis){dyn=dyn, grav=grav}
      mask prompts: dyn "Matriz de parámetros dinámicos:"; grav "Vector aceleración de la gravedad:"
      mask help: Este bloque devuelve el par correspondiente al término de Coriolis.
      mask Help: A este bloque hay que darle tres parámetros: 1) La matriz de parámetros dinámicos del manipulador de acuerdo con el formato que se explica en la sección "dyn" del Apéndice, 2) Un vector columna correspondiente a la aceleración de la gravedad, y 3) Un vector columna correspondiente a las fuerzas externas.
  Términos centrífugos y de Coriolis : Subsystem  mask(Término de Coriolis){dyn=dyn}
      mask prompts: dyn "Matriz de parámetros dinámicos:"
      mask help: Este bloque devuelve el par correspondiente al término de Coriolis.
      mask Help: A este bloque hay que darle tres parámetros: 1) La matriz de parámetros dinámicos del manipulador de acuerdo con el formato que se explica en la sección "dyn" del Apéndice, 2) Un vector columna correspondiente a la aceleración de la gravedad, y 3) Un vector columna correspondiente a las fuerzas externas.
  q : Outport  Port=1  InitialOutput=0
  q' : Outport  Port=2  InitialOutput=0
  q'' : Outport  Port=3  InitialOutput=0
  wires:
  Modelo de fricciones/1(tau_f) -> Sum/2
  Términos centrífugos y de Coriolis/1(V (q,q')) -> Sum/3
  Términos gravitatorios/1(G (q)) -> Sum/4
  Inversa de la matriz de masas/1(M(q)^(-1) · In) -> q''/1, Integrator/1
  tau/1 -> Sum/1
  Sum/1 -> Inversa de la matriz de masas/2(In)
  Integrator/1 -> Modelo de fricciones/1(q'), Términos centrífugos y de Coriolis/2(q'), q'/1, Integrator1/1
  Integrator1/1 -> Términos gravitatorios/1(q), Términos centrífugos y de Coriolis/1(q), Inversa de la matriz de masas/1(q), q/1

== system HEMERO/Robots manipuladores base fija/Modelo Dinámico/Ejemplos/Ejemplo H.4.4a/Inversa de la matriz de masas ==
  q : Inport  Port=1  PortWidth=-1  SampleTime=-1  DataType=auto
      settings: SignalType=auto
  In : Inport  Port=2  PortWidth=-1  SampleTime=-1  DataType=auto
      settings: SignalType=auto
  Masas : S-Function  FunctionName=sminv  Parameters=dyn  PortCounts=[]  SFunctionModules=''
  Mux : Mux  Inputs=2
      settings: DisplayOption=none
  M(q)^(-1) · In : Outport  Port=1  InitialOutput=0
  wires:
  Masas/1 -> M(q)^(-1) · In/1
  In/1 -> Mux/2
  q/1 -> Mux/1
  Mux/1 -> Masas/1

== system HEMERO/Robots manipuladores base fija/Modelo Dinámico/Ejemplos/Ejemplo H.4.4a/Términos gravitatorios ==
  q : Inport  Port=1  PortWidth=-1  SampleTime=-1  DataType=auto
      settings: SignalType=auto
  Gravedad : S-Function  FunctionName=sgravity  Parameters=dyn,grav  PortCounts=[]  SFunctionModules=''
  G (q) : Outport  Port=1  InitialOutput=0
  wires:
  q/1 -> Gravedad/1
  Gravedad/1 -> G (q)/1

== system HEMERO/Robots manipuladores base fija/Modelo Dinámico/Ejemplos/Ejemplo H.4.4a/Términos centrífugos y de Coriolis ==
  q : Inport  Port=1  PortWidth=-1  SampleTime=-1  DataType=auto
      settings: SignalType=auto
  q' : Inport  Port=2  PortWidth=-1  SampleTime=-1  DataType=auto
      settings: SignalType=auto
  Centrífugos y Coriolis : S-Function  FunctionName=scoriolis  Parameters=dyn  PortCounts=[]  SFunctionModules=''
  Mux : Mux  Inputs=2
      settings: DisplayOption=none
  V (q,q') : Outport  Port=1  InitialOutput=0
  wires:
  Mux/1 -> Centrífugos y Coriolis/1
  q/1 -> Mux/1
  q'/1 -> Mux/2
  Centrífugos y Coriolis/1 -> V (q,q')/1

== system HEMERO/Robots manipuladores base fija/Modelo Dinámico/Ejemplos/Ejemplo H.4.4b/Inversa de la matriz de masas ==
  q : Inport  Port=1  PortWidth=-1  SampleTime=-1  DataType=auto
      settings: SignalType=auto
  In : Inport  Port=2  PortWidth=-1  SampleTime=-1  DataType=auto
      settings: SignalType=auto
  Masas : S-Function  FunctionName=sminv  Parameters=dyn  PortCounts=[]  SFunctionModules=''
  Mux : Mux  Inputs=2
      settings: DisplayOption=none
  M(q)^(-1) · In : Outport  Port=1  InitialOutput=0
  wires:
  Masas/1 -> M(q)^(-1) · In/1
  In/1 -> Mux/2
  q/1 -> Mux/1
  Mux/1 -> Masas/1

== system HEMERO/Robots manipuladores base fija/Modelo Dinámico/Ejemplos/Ejemplo H.4.4b/Términos gravitatorios ==
  q : Inport  Port=1  PortWidth=-1  SampleTime=-1  DataType=auto
      settings: SignalType=auto
  Gravedad : S-Function  FunctionName=sgravity  Parameters=dyn,grav  PortCounts=[]  SFunctionModules=''
  G (q) : Outport  Port=1  InitialOutput=0
  wires:
  q/1 -> Gravedad/1
  Gravedad/1 -> G (q)/1

== system HEMERO/Robots manipuladores base fija/Modelo Dinámico/Ejemplos/Ejemplo H.4.4b/Términos centrífugos y de Coriolis ==
  q : Inport  Port=1  PortWidth=-1  SampleTime=-1  DataType=auto
      settings: SignalType=auto
  q' : Inport  Port=2  PortWidth=-1  SampleTime=-1  DataType=auto
      settings: SignalType=auto
  Centrífugos y Coriolis : S-Function  FunctionName=scoriolis  Parameters=dyn  PortCounts=[]  SFunctionModules=''
  Mux : Mux  Inputs=2
      settings: DisplayOption=none
  V (q,q') : Outport  Port=1  InitialOutput=0
  wires:
  Centrífugos y Coriolis/1 -> V (q,q')/1
  q'/1 -> Mux/2
  q/1 -> Mux/1
  Mux/1 -> Centrífugos y Coriolis/1

== system HEMERO/Robots manipuladores base fija/Modelo Dinámico/Ejemplos/Ejemplo H.4.4c/Inversa de la matriz de masas ==
  q : Inport  Port=1  PortWidth=-1  SampleTime=-1  DataType=auto
      settings: SignalType=auto
  In : Inport  Port=2  PortWidth=-1  SampleTime=-1  DataType=auto
      settings: SignalType=auto
  Masas : S-Function  FunctionName=sminv  Parameters=dyn  PortCounts=[]  SFunctionModules=''
  Mux : Mux  Inputs=2
      settings: DisplayOption=none
  M(q)^(-1) · In : Outport  Port=1  InitialOutput=0
  wires:
  Masas/1 -> M(q)^(-1) · In/1
  In/1 -> Mux/2
  q/1 -> Mux/1
  Mux/1 -> Masas/1

== system HEMERO/Robots manipuladores base fija/Modelo Dinámico/Ejemplos/Ejemplo H.4.4c/Modelo de fricciones1 ==
  q' : Inport  Port=1  PortWidth=-1  SampleTime=-1  DataType=auto
      settings: SignalType=auto
  Fricciones : S-Function  FunctionName=sfriction  Parameters=G,b,tcp,tcm  PortCounts=[]  SFunctionModules=''
  tau_f : Outport  Port=1  InitialOutput=0
  wires:
  q'/1 -> Fricciones/1
  Fricciones/1 -> tau_f/1

== system HEMERO/Robots manipuladores base fija/Modelo Dinámico/Ejemplos/Ejemplo H.4.4c/Términos gravitatorios1 ==
  q : Inport  Port=1  PortWidth=-1  SampleTime=-1  DataType=auto
      settings: SignalType=auto
  Gravedad : S-Function  FunctionName=sgravity  Parameters=dyn,grav  PortCounts=[]  SFunctionModules=''
  G (q) : Outport  Port=1  InitialOutput=0
  wires:
  q/1 -> Gravedad/1
  Gravedad/1 -> G (q)/1

== system HEMERO/Robots manipuladores base fija/Modelo Dinámico/Ejemplos/Ejemplo H.4.4c/Términos centrífugos y de Coriolis ==
  q : Inport  Port=1  PortWidth=-1  SampleTime=-1  DataType=auto
      settings: SignalType=auto
  q' : Inport  Port=2  PortWidth=-1  SampleTime=-1  DataType=auto
      settings: SignalType=auto
  Centrífugos y Coriolis : S-Function  FunctionName=scoriolis  Parameters=dyn  PortCounts=[]  SFunctionModules=''
  Mux : Mux  Inputs=2
      settings: DisplayOption=none
  V (q,q') : Outport  Port=1  InitialOutput=0
  wires:
  Centrífugos y Coriolis/1 -> V (q,q')/1
  q'/1 -> Mux/2
  q/1 -> Mux/1
  Mux/1 -> Centrífugos y Coriolis/1

== system HEMERO/Robots móviles/Control de robots móviles/Métodos geométricos/Pure Pursuit I/Cálculo de incremento de x ==
  x_ob : Inport  Port=1  PortWidth=-1  SampleTime=-1  DataType=auto
      settings: SignalType=auto
  y_ob : Inport  Port=2  PortWidth=-1  SampleTime=-1  DataType=auto
      settings: SignalType=auto
  x_vehículo : Inport  Port=3  PortWidth=-1  SampleTime=-1  DataType=auto
      settings: SignalType=auto
  y_vehículo : Inport  Port=4  PortWidth=-1  SampleTime=-1  DataType=auto
      settings: SignalType=auto
  phi_vehículo : Inport  Port=5  PortWidth=-1  SampleTime=-1  DataType=auto
      settings: SignalType=auto
  Product : Product  Inputs=2  SaturateOnIntegerOverflow=on
  Product1 : Product  Inputs=2  SaturateOnIntegerOverflow=on
  Sum : Sum  Inputs=+-  SaturateOnIntegerOverflow=on
  Sum1 : Sum  Inputs=+-  SaturateOnIntegerOverflow=on
  Sum2 : Sum  Inputs=++  SaturateOnIntegerOverflow=on
  Trigonometric Function : Trigonometry  Operator=sin  OutputSignalType=auto
  Trigonometric Function1 : Trigonometry  Operator=cos  OutputSignalType=auto
  incremento_x : Outport  Port=1
  wires:
  x_ob/1 -> Sum/1
  x_vehículo/1 -> Sum/2
  y_ob/1 -> Sum1/1
  y_vehículo/1 -> Sum1/2
  Sum/1 -> Product/1
  Trigonometric Function1/1 -> Product/2
  phi_vehículo/1 -> Trigonometric Function1/1, Trigonometric Function/1
  Sum1/1 -> Product1/1
  Trigonometric Function/1 -> Product1/2
  Product/1 -> Sum2/1
  Product1/1 -> Sum2/2
  Sum2/1 -> incremento_x/1

== system HEMERO/Robots móviles/Control de robots móviles/Métodos geométricos/Pure Pursuit II/Cálculo de L ==
  x_ob : Inport  Port=1  PortWidth=-1  SampleTime=-1  DataType=auto
      settings: SignalType=auto
  y_ob : Inport  Port=2  PortWidth=-1  SampleTime=-1  DataType=auto
      settings: SignalType=auto
  x_vehículo : Inport  Port=3  PortWidth=-1  SampleTime=-1  DataType=auto
      settings: SignalType=auto
  y_vehículo : Inport  Port=4  PortWidth=-1  SampleTime=-1  DataType=auto
      settings: SignalType=auto
  Math Function : Math  Operator=magnitude^2  OutputSignalType=auto
  Math Function1 : Math  Operator=magnitude^2  OutputSignalType=auto
  Math Function2 : Math  Operator=sqrt  OutputSignalType=auto
  Sum : Sum  Inputs=+-  SaturateOnIntegerOverflow=on
  Sum1 : Sum  Inputs=+-  SaturateOnIntegerOverflow=on
  Sum2 : Sum  Inputs=++  SaturateOnIntegerOverflow=on
  L : Outport  Port=1
  wires:
  y_ob/1 -> Sum1/1
  y_vehículo/1 -> Sum1/2
  Sum1/1 -> Math Function1/1
  Math Function1/1 -> Sum2/2
  x_ob/1 -> Sum/1
  x_vehículo/1 -> Sum/2
  Sum/1 -> Math Function/1
  Math Function/1 -> Sum2/1
  Sum2/1 -> Math Function2/1
  Math Function2/1 -> L/1

== system HEMERO/Robots móviles/Control de robots móviles/Métodos geométricos/Pure Pursuit II/Cálculo de incremento de x ==
  x_ob : Inport  Port=1  PortWidth=-1  SampleTime=-1  DataType=auto
      settings: SignalType=auto
  y_ob : Inport  Port=2  PortWidth=-1  SampleTime=-1  DataType=auto
      settings: SignalType=auto
  x_vehículo : Inport  Port=3  PortWidth=-1  SampleTime=-1  DataType=auto
      settings: SignalType=auto
  y_vehículo : Inport  Port=4  PortWidth=-1  SampleTime=-1  DataType=auto
      settings: SignalType=auto
  phi_vehículo : Inport  Port=5  PortWidth=-1  SampleTime=-1  DataType=auto
      settings: SignalType=auto
  Product : Product  Inputs=2  SaturateOnIntegerOverflow=on
  Product1 : Product  Inputs=2  SaturateOnIntegerOverflow=on
  Sum : Sum  Inputs=+-  SaturateOnIntegerOverflow=on
  Sum1 : Sum  Inputs=+-  SaturateOnIntegerOverflow=on
  Sum2 : Sum  Inputs=++  SaturateOnIntegerOverflow=on
  Trigonometric Function : Trigonometry  Operator=sin  OutputSignalType=auto
  Trigonometric Function1 : Trigonometry  Operator=cos  OutputSignalType=auto
  incremento_x : Outport  Port=1
  wires:
  Sum2/1 -> incremento_x/1
  Product1/1 -> Sum2/2
  Product/1 -> Sum2/1
  Trigonometric Function/1 -> Product1/2
  Sum1/1 -> Product1/1
  phi_vehículo/1 -> Trigonometric Function/1, Trigonometric Function1/1
  Trigonometric Function1/1 -> Product/2
  Sum/1 -> Product/1
  y_vehículo/1 -> Sum1/2
  y_ob/1 -> Sum1/1
  x_vehículo/1 -> Sum/2
  x_ob/1 -> Sum/1

== system HEMERO/Robots móviles/Control de robots móviles/Métodos geométricos/Pure Pursuit III/Cálculo de L ==
  x_ob : Inport  Port=1  PortWidth=-1  SampleTime=-1  DataType=auto
      settings: SignalType=auto
  y_ob : Inport  Port=2  PortWidth=-1  SampleTime=-1  DataType=auto
      settings: SignalType=auto
  x_vehículo : Inport  Port=3  PortWidth=-1  SampleTime=-1  DataType=auto
      settings: SignalType=auto
  y_vehículo : Inport  Port=4  PortWidth=-1  SampleTime=-1  DataType=auto
      settings: SignalType=auto
  Math Function : Math  Operator=magnitude^2  OutputSignalType=auto
  Math Function1 : Math  Operator=magnitude^2  OutputSignalType=auto
  Math Function2 : Math  Operator=sqrt  OutputSignalType=auto
  Sum : Sum  Inputs=+-  SaturateOnIntegerOverflow=on
  Sum1 : Sum  Inputs=+-  SaturateOnIntegerOverflow=on
  Sum2 : Sum  Inputs=++  SaturateOnIntegerOverflow=on
  L : Outport  Port=1
  wires:
  Math Function2/1 -> L/1
  Sum2/1 -> Math Function2/1
  Math Function/1 -> Sum2/1
  Sum/1 -> Math Function/1
  x_vehículo/1 -> Sum/2
  x_ob/1 -> Sum/1
  Math Function1/1 -> Sum2/2
  Sum1/1 -> Math Function1/1
  y_vehículo/1 -> Sum1/2
  y_ob/1 -> Sum1/1

== system HEMERO/Robots móviles/Control de robots móviles/Métodos geométricos/Pure Pursuit III/Cálculo de incremento de x ==
  x_ob : Inport  Port=1  PortWidth=-1  SampleTime=-1  DataType=auto
      settings: SignalType=auto
  y_ob : Inport  Port=2  PortWidth=-1  SampleTime=-1  DataType=auto
      settings: SignalType=auto
  x_vehículo : Inport  Port=3  PortWidth=-1  SampleTime=-1  DataType=auto
      settings: SignalType=auto
  y_vehículo : Inport  Port=4  PortWidth=-1  SampleTime=-1  DataType=auto
      settings: SignalType=auto
  phi_vehículo : Inport  Port=5  PortWidth=-1  SampleTime=-1  DataType=auto
      settings: SignalType=auto
  Product : Product  Inputs=2  SaturateOnIntegerOverflow=on
  Product1 : Product  Inputs=2  SaturateOnIntegerOverflow=on
  Sum : Sum  Inputs=+-  SaturateOnIntegerOverflow=on
  Sum1 : Sum  Inputs=+-  SaturateOnIntegerOverflow=on
  Sum2 : Sum  Inputs=++  SaturateOnIntegerOverflow=on
  Trigonometric Function : Trigonometry  Operator=sin  OutputSignalType=auto
  Trigonometric Function1 : Trigonometry  Operator=cos  OutputSignalType=auto
  incremento_x : Outport  Port=1
  wires:
  x_ob/1 -> Sum/1
  x_vehículo/1 -> Sum/2
  y_ob/1 -> Sum1/1
  y_vehículo/1 -> Sum1/2
  Sum/1 -> Product/1
  Trigonometric Function1/1 -> Product/2
  phi_vehículo/1 -> Trigonometric Function1/1, Trigonometric Function/1
  Sum1/1 -> Product1/1
  Trigonometric Function/1 -> Product1/2
  Product/1 -> Sum2/1
  Product1/1 -> Sum2/2
  Sum2/1 -> incremento_x/1

== system HEMERO/Robots móviles/Control de robots móviles/Métodos basados en Teoría de Control/Seguimiento de caminos/Ejemplos ==
  Ejemplo H.6.4 : Subsystem
  Ejemplo H.6.5 : Subsystem
